simulink model "nelin_sim"  (R2020a)
settings: Solver=ode5  StartTime=0.0  StopTime=tfin  FixedStep=1e-4  RelTol=1e-3
values from neighbouring files (symbols this model uses):
  F = Fe    [nelin_sim_matlab.m]
  F_step1 = 0    [nelin_sim_matlab.m]
  F_step2 = Fe    [nelin_sim_matlab.m]
  Fe = double(mi_Se*V)    [nelin_sim_matlab.m]
  K1 = 0.03    [nelin_sim_matlab.m]
  K2 = 0.5    [nelin_sim_matlab.m]
  mi_max = 1    [nelin_sim_matlab.m]
  Se = Ses(2)    [nelin_sim_matlab.m]
  SF = 10    [nelin_sim_matlab.m]
  tF_step1 = 2    [nelin_sim_matlab.m]
  tF_step2 = 5    [nelin_sim_matlab.m]
  V = 4    [nelin_sim_matlab.m]
  x10 = Xe    [nelin_sim_matlab.m]
  x20 = Se    [nelin_sim_matlab.m]
  Y = 0.5    [nelin_sim_matlab.m]
undefined symbols (not defined in the file or in its folder): A, B, C, magnitude
settings Model: Creator=anaMceranic  LastModifiedBy=anaMceranic
settings DataIOCC: ReturnWorkspaceOutputs=off

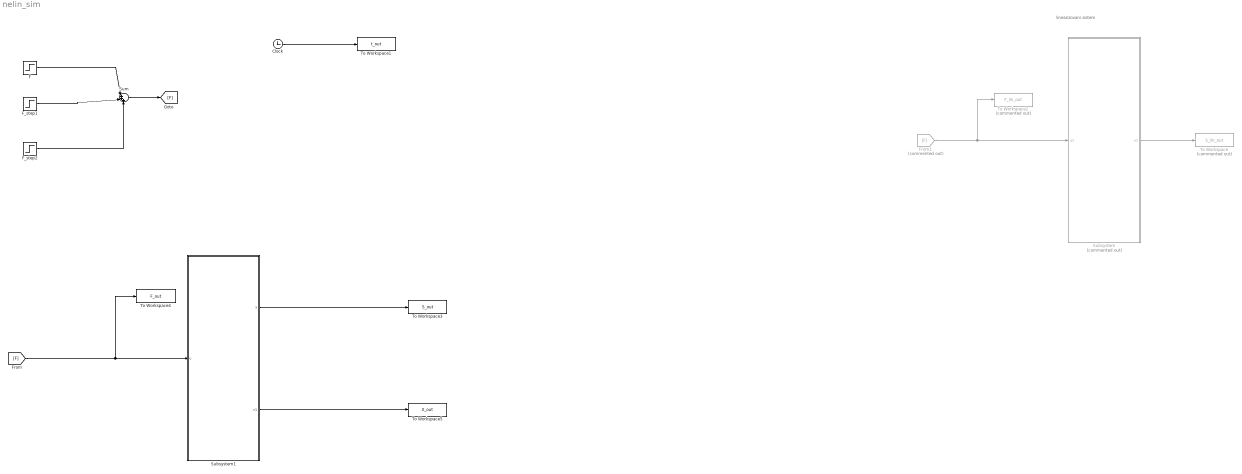
== system nelin_sim ==
  note: linearizovani sistem
  Clock : Clock
  F : Step  Time=0  Before=F  After=F  SampleTime=0
  F_step1 : Step  Time=tF_step1  After=F_step1  SampleTime=0
  F_step2 : Step  Time=tF_step2  After=-F_step2  SampleTime=0
  From1 : From  Commented=on  GotoTag=F
  Subsystem : Subsystem  Commented=on
  Subsystem1 : Subsystem
  Sum : Sum  Inputs=|+++
  To Workspace : ToWorkspace  Commented=on  VariableName=S_lin_out  SampleTime=-1
  To Workspace1 : ToWorkspace  VariableName=t_out  SampleTime=-1
  To Workspace2 : ToWorkspace  Commented=on  VariableName=F_lin_out  SampleTime=-1
  To Workspace3 : ToWorkspace  VariableName=S_out  SampleTime=-1
  To Workspace4 : ToWorkspace  VariableName=F_out  SampleTime=-1
  To Workspace5 : ToWorkspace  VariableName=X_out  SampleTime=-1
  wires:
  Subsystem/1(y1) -> To Workspace/1
  Clock/1 -> To Workspace1/1
  F/1 -> Sum/1
  F_step1/1 -> Sum/2
  F_step2/1 -> Sum/3
  Sum/1 -> [F]
  From1/1 -> To Workspace2/1, Subsystem/1(u1)
  [F] -> To Workspace4/1, Subsystem1/1(u)
  Subsystem1/1(y) -> To Workspace3/1
  Subsystem1/2(x1) -> To Workspace5/1

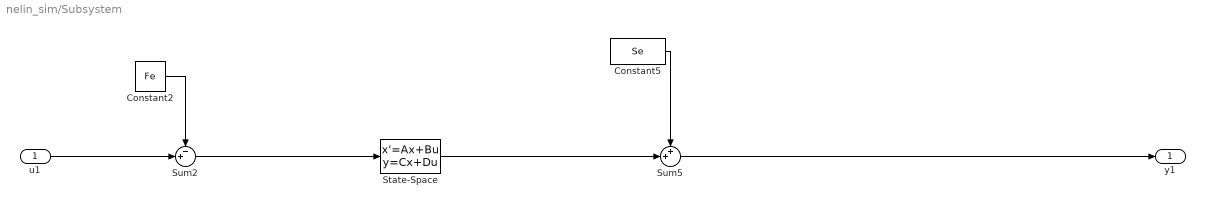
== system nelin_sim/Subsystem ==
  u1 : Inport
  Constant2 : Constant  Value=Fe
  Constant5 : Constant  Value=Se
  State-Space : StateSpace  A=A  B=B  C=C  D=[0]  InitialCondition=0
  Sum2 : Sum  Inputs=-+|
  Sum5 : Sum  Inputs=++|
  y1 : Outport
  wires:
  Constant5/1 -> Sum5/1
  Sum5/1 -> y1/1
  State-Space/1 -> Sum5/2
  Sum2/1 -> State-Space/1
  Constant2/1 -> Sum2/1
  u1/1 -> Sum2/2

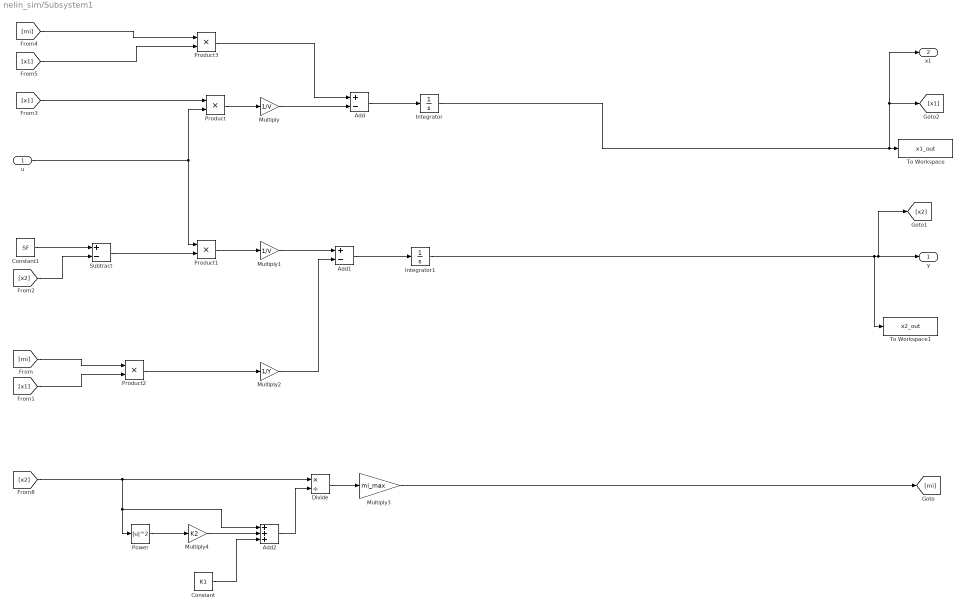
== system nelin_sim/Subsystem1 ==
  u : Inport
  Add : Sum  Inputs=+-
  Add1 : Sum  Inputs=+-
  Add2 : Sum  Inputs=+++
  Constant : Constant  Value=K1
  Constant1 : Constant  Value=SF
  Divide : Product  Inputs=*/
  Integrator : Integrator  InitialCondition=x10
  Integrator1 : Integrator  InitialCondition=x20
  Multiply : Gain  Gain=1/V
  Multiply1 : Gain  Gain=1/V
  Multiply2 : Gain  Gain=1/Y
  Multiply3 : Gain  Gain=mi_max
  Multiply4 : Gain  Gain=K2
  Power : Math  Operator=magnitude^2  SaturateOnIntegerOverflow=on
  Product{,1..3} (4 alike) : Product
  Subtract : Sum  Inputs=+-
  To Workspace : ToWorkspace  VariableName=x1_out  SampleTime=-1
  To Workspace1 : ToWorkspace  VariableName=x2_out  SampleTime=-1
  y : Outport
  x1 : Outport  Port=2
  wires:
  [x1] -> Product2/2
  Product2/1 -> Multiply2/1
  Multiply/1 -> Add/2
  Add2/1 -> Divide/2
  Constant/1 -> Add2/3
  [x1] -> Product3/2
  Multiply4/1 -> Add2/2
  [mi] -> Product2/1
  Multiply3/1 -> [mi]
  Power/1 -> Multiply4/1
  Constant1/1 -> Subtract/1
  [x2] -> Subtract/2
  Add1/1 -> Integrator1/1
  Multiply2/1 -> Add1/2
  Integrator1/1 -> [x2], y/1, To Workspace1/1
  Divide/1 -> Multiply3/1
  Product3/1 -> Add/1
  u/1 -> Product1/1, Product/2
  [x1] -> Product/1
  Multiply1/1 -> Add1/1
  Product1/1 -> Multiply1/1
  Subtract/1 -> Product1/2
  [x2] -> Divide/1, Add2/1, Power/1
  Add/1 -> Integrator/1
  Product/1 -> Multiply/1
  [mi] -> Product3/1
  Integrator/1 -> [x1], x1/1, To Workspace/1
